simulink model "CubeX_Fast_MPC_2D"  (R2016b)
settings: Solver=FixedStepDiscrete  StartTime=0.0  StopTime=inf  FixedStep=Ts.base  RelTol=1e-3
PreLoadFcn:
  | waijung.modelPreload; % Required for working with Waijung Blockset. Do not remove.
InitFcn:
  | cubeparameters
undefined symbols (not defined in the file or in its folder): CPHA_1Edge, CPOL_Low, deg_, Duplex, FirstBit_MSB, Full, g, imu, Link, LQFP100, ST, STM32F407VG, STM32F4DISCOVERY, Ts
libraries: simulink x47, stm32f4_i2c_lib x12, stm32f4_io_lib x5, stm32f4_spi_lib x4, cube_lib x3, BC_USB x2, stm32f4_adc_lib x1, stm32f4_device_config_lib x1
(part 3 of 3)

== system CubeX_Fast_MPC_2D/Read IMU/Magnetometer I2C1/AK8963 Init /Write Configuration ==
  SlvAddr : Inport
  RegAddr : Inport  Port=2
  Enable : EnablePort
  I2C Master Read/Write1 : stm32f4_i2c_lib/I2C Master Read//Write  configuration=Transaction  module=1  lastmodule=3  transfer=Blocking  dutycycle=TLow/THigh = 2  clkspeed=400  timeout=25  writecount=2  readcount=0  sdapin=C9  sclpin=A8  waitwritetime=0  forcestop=off  inputtypearray=[3 3 3 3]  outputtypearray=[1 3]  confstr="[\"C\",\"9\",\"A\",\"8\",\"1\",\"1\",\"6\",\"0\",\"I2C_DutyCycle_2\",\"0\",\"off\"]"  sampletime=-1  sampletimestr=0.002  blockid=ReadIMUMagnetometerI2CAK8963InitWriteConfigurationI2CMasterReadWrite1
  Terminator : Terminator
  "bit[5] : 16-bit output bit[3:0] - Continuous measurement mode 2" : Constant  Value=hex2dec('16')  OutDataTypeStr=uint8  SampleTime=-1
  wires:
  RegAddr/1 -> I2C Master Read/Write1/2
  SlvAddr/1 -> I2C Master Read/Write1/1
  I2C Master Read/Write1/1 -> Terminator/1
  "bit[5] : 16-bit output bit[3:0] - Continuous measurement mode 2"/1 -> I2C Master Read/Write1/3

== system CubeX_Fast_MPC_2D/Read IMU/Magnetometer I2C1/Read Magnetometer Data/Turn the MSB and LSB into a signed 16-bit integer MagX ==
  low : Inport
  high : Inport  Port=2
  Bitwise Operator2 : simulink/Logic and Bit Operations/Bitwise Operator  logicop=OR  UseBitMask=off  NumInputPorts=2  BitMask=bin2dec('11011001')  BitMaskRealWorld=Stored Integer
  Data Type Conversion6 : DataTypeConversion  OutDataTypeStr=uint16
  Data Type Conversion7 : DataTypeConversion  OutDataTypeStr=uint16
  Shift Arithmetic2 : ArithShift  BitShiftNumber=-8
  out16b : Outport
  wires:
  low/1 -> Data Type Conversion6/1
  Bitwise Operator2/1 -> out16b/1
  high/1 -> Data Type Conversion7/1
  Data Type Conversion7/1 -> Shift Arithmetic2/1
  Shift Arithmetic2/1 -> Bitwise Operator2/2
  Data Type Conversion6/1 -> Bitwise Operator2/1

== system CubeX_Fast_MPC_2D/Read IMU/Magnetometer I2C1/Read Magnetometer Data/Turn the MSB and LSB into a signed 16-bit integer MagY ==
  low : Inport
  high : Inport  Port=2
  Bitwise Operator2 : simulink/Logic and Bit Operations/Bitwise Operator  logicop=OR  UseBitMask=off  NumInputPorts=2  BitMask=bin2dec('11011001')  BitMaskRealWorld=Stored Integer
  Data Type Conversion6 : DataTypeConversion  OutDataTypeStr=uint16
  Data Type Conversion7 : DataTypeConversion  OutDataTypeStr=uint16
  Shift Arithmetic2 : ArithShift  BitShiftNumber=-8
  out16b : Outport
  wires:
  low/1 -> Data Type Conversion6/1
  Bitwise Operator2/1 -> out16b/1
  high/1 -> Data Type Conversion7/1
  Data Type Conversion7/1 -> Shift Arithmetic2/1
  Shift Arithmetic2/1 -> Bitwise Operator2/2
  Data Type Conversion6/1 -> Bitwise Operator2/1

== system CubeX_Fast_MPC_2D/Read IMU/Magnetometer I2C1/Read Magnetometer Data/Turn the MSB and LSB into a signed 16-bit integer MagZ ==
  low : Inport
  high : Inport  Port=2
  Bitwise Operator2 : simulink/Logic and Bit Operations/Bitwise Operator  logicop=OR  UseBitMask=off  NumInputPorts=2  BitMask=bin2dec('11011001')  BitMaskRealWorld=Stored Integer
  Data Type Conversion6 : DataTypeConversion  OutDataTypeStr=uint16
  Data Type Conversion7 : DataTypeConversion  OutDataTypeStr=uint16
  Shift Arithmetic2 : ArithShift  BitShiftNumber=-8
  out16b : Outport
  wires:
  low/1 -> Data Type Conversion6/1
  Bitwise Operator2/1 -> out16b/1
  high/1 -> Data Type Conversion7/1
  Data Type Conversion7/1 -> Shift Arithmetic2/1
  Shift Arithmetic2/1 -> Bitwise Operator2/2
  Data Type Conversion6/1 -> Bitwise Operator2/1

== system CubeX_Fast_MPC_2D/Read IMU/Accelometer Gyroscope I2C1/Read Accelometer and Gyroscope Data/Old gyro get data Used during SPI before/USE THIS ONE!!2 ==
  "Gyro_Zout_High " : Inport
  Gyro_Zout_Low : Inport  Port=2
  Bitwise Operator : simulink/Logic and Bit Operations/Bitwise Operator  logicop=OR  UseBitMask=off  NumInputPorts=2  BitMask=bin2dec('11011001')  BitMaskRealWorld=Stored Integer
  Data Type Conversion : DataTypeConversion  OutDataTypeStr=uint16
  Data Type Conversion1 : DataTypeConversion  OutDataTypeStr=uint16
  Shift Arithmetic : ArithShift  BitShiftNumber=-8
  Gyro_Zout : Outport
  wires:
  Gyro_Zout_Low/1 -> Data Type Conversion/1
  "Gyro_Zout_High "/1 -> Data Type Conversion1/1
  Data Type Conversion1/1 -> Shift Arithmetic/1
  Data Type Conversion/1 -> Bitwise Operator/2
  Shift Arithmetic/1 -> Bitwise Operator/1
  Bitwise Operator/1 -> Gyro_Zout/1

== system CubeX_Fast_MPC_2D/Read IMU/Accelometer Gyroscope I2C1/Read Accelometer and Gyroscope Data/Old gyro get data Used during SPI before/USE THIS ONE!!3 ==
  "Gyro_Zout_High " : Inport
  Gyro_Zout_Low : Inport  Port=2
  Bitwise Operator : simulink/Logic and Bit Operations/Bitwise Operator  logicop=OR  UseBitMask=off  NumInputPorts=2  BitMask=bin2dec('11011001')  BitMaskRealWorld=Stored Integer
  Data Type Conversion : DataTypeConversion  OutDataTypeStr=uint16
  Data Type Conversion1 : DataTypeConversion  OutDataTypeStr=uint16
  Shift Arithmetic : ArithShift  BitShiftNumber=-8
  Gyro_Zout : Outport
  wires:
  Gyro_Zout_Low/1 -> Data Type Conversion/1
  "Gyro_Zout_High "/1 -> Data Type Conversion1/1
  Data Type Conversion1/1 -> Shift Arithmetic/1
  Data Type Conversion/1 -> Bitwise Operator/2
  Shift Arithmetic/1 -> Bitwise Operator/1
  Bitwise Operator/1 -> Gyro_Zout/1

== system CubeX_Fast_MPC_2D/Read IMU/Accelometer Gyroscope I2C1/Read Accelometer and Gyroscope Data/Old gyro get data Used during SPI before/USE THIS ONE!!4 ==
  "Gyro_Zout_High " : Inport
  Gyro_Zout_Low : Inport  Port=2
  Bitwise Operator : simulink/Logic and Bit Operations/Bitwise Operator  logicop=OR  UseBitMask=off  NumInputPorts=2  BitMask=bin2dec('11011001')  BitMaskRealWorld=Stored Integer
  Data Type Conversion : DataTypeConversion  OutDataTypeStr=uint16
  Data Type Conversion1 : DataTypeConversion  OutDataTypeStr=uint16
  Shift Arithmetic : ArithShift  BitShiftNumber=-8
  Gyro_Zout : Outport
  wires:
  Gyro_Zout_Low/1 -> Data Type Conversion/1
  "Gyro_Zout_High "/1 -> Data Type Conversion1/1
  Data Type Conversion1/1 -> Shift Arithmetic/1
  Data Type Conversion/1 -> Bitwise Operator/2
  Shift Arithmetic/1 -> Bitwise Operator/1
  Bitwise Operator/1 -> Gyro_Zout/1

== system CubeX_Fast_MPC_2D/Read IMU/Accelometer Gyroscope I2C3/Read Accelometer and Gyroscope Data/Old gyro get data Used during SPI before/USE THIS ONE!!2 ==
  "Gyro_Zout_High " : Inport
  Gyro_Zout_Low : Inport  Port=2
  Bitwise Operator : simulink/Logic and Bit Operations/Bitwise Operator  logicop=OR  UseBitMask=off  NumInputPorts=2  BitMask=bin2dec('11011001')  BitMaskRealWorld=Stored Integer
  Data Type Conversion : DataTypeConversion  OutDataTypeStr=uint16
  Data Type Conversion1 : DataTypeConversion  OutDataTypeStr=uint16
  Shift Arithmetic : ArithShift  BitShiftNumber=-8
  Gyro_Zout : Outport
  wires:
  Gyro_Zout_Low/1 -> Data Type Conversion/1
  "Gyro_Zout_High "/1 -> Data Type Conversion1/1
  Data Type Conversion1/1 -> Shift Arithmetic/1
  Data Type Conversion/1 -> Bitwise Operator/2
  Shift Arithmetic/1 -> Bitwise Operator/1
  Bitwise Operator/1 -> Gyro_Zout/1

== system CubeX_Fast_MPC_2D/Read IMU/Accelometer Gyroscope I2C3/Read Accelometer and Gyroscope Data/Old gyro get data Used during SPI before/USE THIS ONE!!3 ==
  "Gyro_Zout_High " : Inport
  Gyro_Zout_Low : Inport  Port=2
  Bitwise Operator : simulink/Logic and Bit Operations/Bitwise Operator  logicop=OR  UseBitMask=off  NumInputPorts=2  BitMask=bin2dec('11011001')  BitMaskRealWorld=Stored Integer
  Data Type Conversion : DataTypeConversion  OutDataTypeStr=uint16
  Data Type Conversion1 : DataTypeConversion  OutDataTypeStr=uint16
  Shift Arithmetic : ArithShift  BitShiftNumber=-8
  Gyro_Zout : Outport
  wires:
  Gyro_Zout_Low/1 -> Data Type Conversion/1
  "Gyro_Zout_High "/1 -> Data Type Conversion1/1
  Data Type Conversion1/1 -> Shift Arithmetic/1
  Data Type Conversion/1 -> Bitwise Operator/2
  Shift Arithmetic/1 -> Bitwise Operator/1
  Bitwise Operator/1 -> Gyro_Zout/1

== system CubeX_Fast_MPC_2D/Read IMU/Accelometer Gyroscope I2C3/Read Accelometer and Gyroscope Data/Old gyro get data Used during SPI before/USE THIS ONE!!4 ==
  "Gyro_Zout_High " : Inport
  Gyro_Zout_Low : Inport  Port=2
  Bitwise Operator : simulink/Logic and Bit Operations/Bitwise Operator  logicop=OR  UseBitMask=off  NumInputPorts=2  BitMask=bin2dec('11011001')  BitMaskRealWorld=Stored Integer
  Data Type Conversion : DataTypeConversion  OutDataTypeStr=uint16
  Data Type Conversion1 : DataTypeConversion  OutDataTypeStr=uint16
  Shift Arithmetic : ArithShift  BitShiftNumber=-8
  Gyro_Zout : Outport
  wires:
  Gyro_Zout_Low/1 -> Data Type Conversion/1
  "Gyro_Zout_High "/1 -> Data Type Conversion1/1
  Data Type Conversion1/1 -> Shift Arithmetic/1
  Data Type Conversion/1 -> Bitwise Operator/2
  Shift Arithmetic/1 -> Bitwise Operator/1
  Bitwise Operator/1 -> Gyro_Zout/1

== matlab function CubeX_Fast_MPC_2D/MPC/Fast MPC ==
  data: phi input; iref output size=1; omega input; fMPC parameter; amountIter output
function [iref, amountIter] = fcn(phi,omega, fMPC)

    persistent lamda w

    if isempty(lamda)   
        lamda = zeros(60, 10,'single');    
        w = zeros(90,1,'single');
    end

    xk = [phi ; omega];
    d = fMPC.dd * xk;
    sig = fMPC.LP * d;
    k = single(2);
    while (k < 10) 
        beta = (k-3)/k;
        mu = lamda(:,k) + beta*(lamda(:,k)-lamda(:,k-1));
        KK = [fMPC.inCo fMPC.miHDtPt*mu];
        w = median(KK,2);
        lamda(:,k+1) = mu + (fMPC.LPD * w) - sig;  

        if norm((fMPC.D*w)-d,inf) <= 1e-4
            lamda(:,1:2) = lamda(:,k:k+1);
            break;
        end
        k = k + 1;
    end
    iref = w(1);
    amountIter = k-1;

== matlab function CubeX_Fast_MPC_2D/Read IMU/Rotation of IMU1 ==
  data: acc input; acc_out output; gyro input; gyro_out output; imu parameter
function [acc_out,gyro_out] = fcn(acc,gyro, imu)

acc_out     = imu.rot_IMU1 * single(acc);
gyro_out    = imu.rot_IMU1 * single(gyro);

== matlab function CubeX_Fast_MPC_2D/Read IMU/Magdwick Filter ==
  data: acc input single size=[1 3]; euler output single; gyro input size=[1 3]; Ts parameter
function euler = Magdwick(acc, gyro, Ts)

    persistent AHRS;
    
    if isempty(AHRS)      
       AHRS = MadgwickAHRS('SamplePeriod', Ts.IMU, 'Beta', 0.04); 
    end
    
    AHRS.UpdateIMU(gyro, acc);
    
    q = AHRS.Quaternion;
    euler = quatern2euler(quaternConj(q));

== matlab function CubeX_Fast_MPC_2D/Reference calibration from buttons/Reference calibration calculation ==
  data: ref_plus input; correction_out output; ref_minus input; inital_offset input
function correction_out = ReferenceCalibration(ref_plus,ref_minus,inital_offset)
%#codegen

persistent correction;

delta_correction = 0.01; % NOTE: Degrees!

if isempty(correction)
    correction = inital_offset;   % Initial calibration is estimated center of gravity offset from geometrical center, in degrees.
end

if ref_plus == true
    correction = correction + delta_correction;
end

if ref_minus == true
    correction = correction - delta_correction;
end

correction_out = correction;

== matlab function CubeX_Fast_MPC_2D/MPC/Estimate COG LP ==
  data Ts settings: description=Sample time for LQR
  data: iref input; phi input; y output size=1; wx input; Ts parameter; wx_l output
function [y ,wx_l]  = fcn(iref, phi, wx, Ts)
%#codegen

%Function that estimates how many the degrees the COG is offset from the
%symmetry line of the cube. 


persistent iref_lp L_COG k_min k phi_offs wx_lp WXL_COG

if(isempty(iref_lp))
   iref_lp = zeros(1,1,'single');
   Tf_COG = single(0.2);              % Time Constant % 2 % Freq
   L_COG  = Ts.controller/(Tf_COG + Ts.controller);  % Filter gain
   phi_offs = zeros(1,1,'single');
   Tmin = single(0.2);                 %Wait at least this long before incrementing
   k_min = single(round(Tmin/Ts.controller)); 
   k = zeros(1,1,'single');
   wx_lp = zeros(1,1,'single');
   wx_tf = single(0.5);              % Time Constant % 0.04
   WXL_COG  = Ts.controller/(wx_tf + Ts.controller);  % Filter gain
end

%is increased by the same angular rate [rad/s] no matter what Ts is
%chosen

c = -0.007*Ts.controller;       %0.005

wx_lp = (1-WXL_COG) * wx_lp + (WXL_COG * wx);
if( abs(wx_lp) < 6e-3 && abs(phi) < deg2rad(2) )   
    k = k + 1;
    
    iref_lp = (1-L_COG) * iref_lp + L_COG * iref;   
    phi_offs = phi_offs + c*iref_lp; 
    if(k > k_min)        
      % iref_lp = iref_lp/(k_min+1); 
        
       k = zeros(1,1,'single'); 
    end
    
else
    k = zeros(1,1,'single');
    %iref_lp = zeros(1,1,'single');  
end
wx_l = wx_lp;
y = phi_offs;

== matlab function CubeX_Fast_MPC_2D/Read IMU/Steady State Kalman Filter ==
  data: gyro input; kf_gyro output
function kf_gyro = fcn(gyro)

persistent gyroFilter;

K = 0.1;

%init
if isempty(gyroFilter)
    gyroFilter = 0;
end

% Steady State Kalman Filter
gyroFilter = gyroFilter + K*(gyro(1) - (gyroFilter));

kf_gyro = [gyroFilter ; 0 ; 0];

== matlab function CubeX_Fast_MPC_2D/Read IMU/LP filter ==
  data: filter_acc output; acc input; gyro input; filter_gyro output
function [filter_acc,filter_gyro] = fcn(acc,gyro)

persistent f_gyro;
persistent f_acc;
persistent L_acc;
persistent L_gyro;


if isempty(f_gyro)
   f_gyro = zeros(3,1);
   f_acc  = zeros(3,1);
   Ts = 0.002;         % Sampling time
   Tf_gyro = 0.035;         % Time Constant % 0.01
   Tf_acc = 0.05;         % Time Constant % 0.05
   L_acc  = Ts/(Tf_acc + Ts);  % Filter gain
   L_gyro  = Ts/(Tf_gyro + Ts);  % Filter gain
end

% LP Filter
f_gyro = (1-L_gyro) * f_gyro + L_gyro * gyro;
f_acc  = (1-L_acc) * f_acc  + L_acc * acc;

filter_gyro = f_gyro;
filter_acc = f_acc;

== matlab function CubeX_Fast_MPC_2D/Read IMU/Moving Average filter MAF ==
  data: angle input; MAF_phi output
function MAF_phi = fcn(angle)

persistent buffer k_samples;
buffer_size = 40; %Length of filter & DEBUG 2 Seems to work
if isempty(buffer)   
    buffer = zeros(buffer_size,1);
    k_samples = 1;
end
    
buffer(k_samples,1) = angle(1);
k_samples = k_samples + 1;

if (k_samples > buffer_size)
    k_samples = 1 ;
end

MAF_phi = [mean(buffer) ; angle(2) ; angle(3) ];

== matlab function CubeX_Fast_MPC_2D/Read IMU/Lp Filter ==
  data: gyro input; filter_gyro output; Ts parameter
function filter_gyro  = fcn(gyro, Ts)

persistent f_gyro;
persistent L_gyro;


if isempty(f_gyro)
   f_gyro = zeros(3,1,'single');
   
   Tf_gyro = single(0.008);              % Time Constant % 0.04
   L_gyro  = Ts.IMU/(Tf_gyro + Ts.IMU);  % Filter gain
end

% LP Filter
f_gyro = (1-L_gyro) * f_gyro + L_gyro * gyro;
filter_gyro = single(f_gyro);

== matlab function CubeX_Fast_MPC_2D/MPC/Estimate COG offset ==
  data Ts settings: description=Sample time for LQR
  data: iref input; phi input; y output size=1; wx input; Ts parameter
function y = fcn(iref, phi, wx, Ts)
%#codegen

%Function that estimates how many the degrees the COG is offset from the
%symmetry line of the cube. 


persistent phi_offs k_min k iref_mean 

if(isempty(phi_offs))
   phi_offs = zeros(1,1,'single');
   Tmin = single(0.4);                 %Wait at least this long before incrementing
   k_min = single(round(Tmin/Ts.controller)); 
   k = zeros(1,1,'single');  
   iref_mean = zeros(1,1,'single'); 
end

%Tuning factor, normalized to the sampling speed of the algoritmh so phi 
%is increased by the same angular rate [rad/s] no matter what Ts is
%chosen
c = -0.19*Ts.controller;
%c=0;

%Wait k_min sample in a stable area before deciding to to anything 
if( abs(wx) < 0.03 && abs(phi) < deg2rad(2) ) 
    k = k + 1; 
    iref_mean = iref_mean + iref; 
    
    if(k > k_min)        
       iref_mean = iref_mean/(k_min+1); 
       phi_offs = phi_offs + c*iref_mean;  
       k = zeros(1,1,'single'); 
       iref_mean = zeros(1,1,'single'); 
    end
    
else
    iref_mean = zeros(1,1,'single');  
    k = zeros(1,1,'single'); 
end

if abs(phi_offs) > 0.8726 % 50 degress
    phi_offs = zeros(1,1,'single');
end
y = phi_offs;

== matlab function CubeX_Fast_MPC_2D/Read IMU/Accelometer Gyroscope I2C3/Read Accelometer and Gyroscope Data/Old gyro get data Used during SPI before/Take away Sensor fail reading ==
  data: y output; new input; old input
function y = fcn(new, old)
%#codegen
if(new > -257 && new < -200)
   y = old;
else
    y = new;
end

== matlab function CubeX_Fast_MPC_2D/Read IMU/Accelometer Gyroscope I2C3/Read Accelometer and Gyroscope Data/Old gyro get data Used during SPI before/Take away Sensor fail reading if two bad in raw ==
  data: y output; new input; old input
function y = fcn(new, old)
%#codegen
if(new > -257 && new < -200)
   y = old;
else
    y = new;
end

== matlab function CubeX_Fast_MPC_2D/Read IMU/Accelometer Gyroscope I2C3/Read Accelometer and Gyroscope Data/Old gyro get data Used during SPI before/Take away Sensor fail reading if two bad in raw1 ==
  data: y output; new input; old input
function y = fcn(new, old)
%#codegen
if(new > -257 && new < -200)
   y = old;
else
    y = new;
end

== matlab function CubeX_Fast_MPC_2D/Read IMU/Accelometer Gyroscope I2C3/Read Accelometer and Gyroscope Data/Old gyro get data Used during SPI before/Take away Sensor fail reading if two bad in raw2 ==
  data: y output; new input; old input
function y = fcn(new, old)
%#codegen
if(new > -257 && new < -200)
   y = old;
else
    y = new;
end

== matlab function CubeX_Fast_MPC_2D/Read IMU/Accelometer Gyroscope I2C3/Read Accelometer and Gyroscope Data/Old gyro get data Used during SPI before/Take away Sensor fail reading1 ==
  data: y output; new input; old input
function y = fcn(new, old)
%#codegen
if(new > -257 && new < -200)
   y = old;
else
    y = new;
end

== matlab function CubeX_Fast_MPC_2D/Read IMU/Accelometer Gyroscope I2C3/Read Accelometer and Gyroscope Data/Old gyro get data Used during SPI before/Take away Sensor fail reading2 ==
  data: y output; new input; old input
function y = fcn(new, old)
%#codegen
if(new > -257 && new < -200)
   y = old;
else
    y = new;
end

== matlab function CubeX_Fast_MPC_2D/Read IMU/Rotation of IMU3 ==
  data: acc input; acc_out output; gyro input; gyro_out output; imu parameter
function [acc_out,gyro_out] = fcn(acc,gyro, imu)

acc_out     = imu.rot_IMU3 * single(acc);
gyro_out    = imu.rot_IMU3 * single(gyro);

== matlab function CubeX_Fast_MPC_2D/Read IMU/Bias Estimation IMU3 ==
  data: gyro input single; gyro_out output
function gyro_out = bias_estimation(gyro)

% For know we only use gyro around x, thus bias estimation for know is only
% on that measurment

persistent w_IMU;
persistent w_bias_IMU;
persistent bias_samples_IMU;

n_samples = 125;

% init
if isempty(w_IMU)
    w_IMU = zeros(3,n_samples,'single');
    w_bias_IMU = zeros(3,1,'single');
    bias_samples_IMU = 1;
end

% Take measurment for one second
if bias_samples_IMU < n_samples
    w_IMU(:,bias_samples_IMU) = gyro;       % Save all measurment in a vector
    bias_samples_IMU = bias_samples_IMU + 1;    % Increase counter
    gyro_out = zeros(3,1,'single');                 % Set output equal to zero

% After n_samples of measurement
elseif bias_samples_IMU == n_samples        
    w_bias_IMU  = mean(w_IMU,2,'native');                % Calculate the mean of the measurment
    bias_samples_IMU = bias_samples_IMU + 1;    % Increase counter
    gyro_out = gyro - w_bias_IMU;                % Set output equal to zero
    
% When bias is cauclauted
else
    gyro_out = gyro - w_bias_IMU;    % Subtract the bias from measurment
end

== matlab function CubeX_Fast_MPC_2D/Read IMU/Accelometer Gyroscope I2C1/Read Accelometer and Gyroscope Data/Old gyro get data Used during SPI before/Take away Sensor fail reading ==
  data: y output; new input; old input
function y = fcn(new, old)
%#codegen
if(new > -257 && new < -200)
   y = old;
else
    y = new;
end

== matlab function CubeX_Fast_MPC_2D/Read IMU/Accelometer Gyroscope I2C1/Read Accelometer and Gyroscope Data/Old gyro get data Used during SPI before/Take away Sensor fail reading if two bad in raw ==
  data: y output; new input; old input
function y = fcn(new, old)
%#codegen
if(new > -257 && new < -200)
   y = old;
else
    y = new;
end

== matlab function CubeX_Fast_MPC_2D/Read IMU/Accelometer Gyroscope I2C1/Read Accelometer and Gyroscope Data/Old gyro get data Used during SPI before/Take away Sensor fail reading if two bad in raw1 ==
  data: y output; new input; old input
function y = fcn(new, old)
%#codegen
if(new > -257 && new < -200)
   y = old;
else
    y = new;
end

== matlab function CubeX_Fast_MPC_2D/Read IMU/Accelometer Gyroscope I2C1/Read Accelometer and Gyroscope Data/Old gyro get data Used during SPI before/Take away Sensor fail reading1 ==
  data: y output; new input; old input
function y = fcn(new, old)
%#codegen
if(new > -257 && new < -200)
   y = old;
else
    y = new;
end

== matlab function CubeX_Fast_MPC_2D/Read IMU/Accelometer Gyroscope I2C1/Read Accelometer and Gyroscope Data/Old gyro get data Used during SPI before/Take away Sensor fail reading if two bad in raw2 ==
  data: y output; new input; old input
function y = fcn(new, old)
%#codegen
if(new > -257 && new < -200)
   y = old;
else
    y = new;
end

== matlab function CubeX_Fast_MPC_2D/Read IMU/Accelometer Gyroscope I2C1/Read Accelometer and Gyroscope Data/Old gyro get data Used during SPI before/Take away Sensor fail reading2 ==
  data: y output; new input; old input
function y = fcn(new, old)
%#codegen
if(new > -257 && new < -200)
   y = old;
else
    y = new;
end
